simulink model "RLCbac2"  (Simulink 8.5)
settings: Solver=ode3  StartTime=0.0  StopTime=10.0  FixedStep=0.1  RelTol=1e-3
settings Model: Creator=ASUS  LastModifiedBy=ASUS
settings DataIOCC: SignalLoggingSaveFormat=Dataset
settings OptimizationCC: ExpressionDepthLimit=128
settings DebuggingCC: UnderspecifiedInitializationDetection=Simplified  MergeDetectMultiDrivingBlocksExec=error  FcnCallInpInsideContextMsg=EnableAllAsError  StateNameClashWarn=none
settings GRTTargetCC: CombineOutputUpdateFcns=on  GRTInterface=off

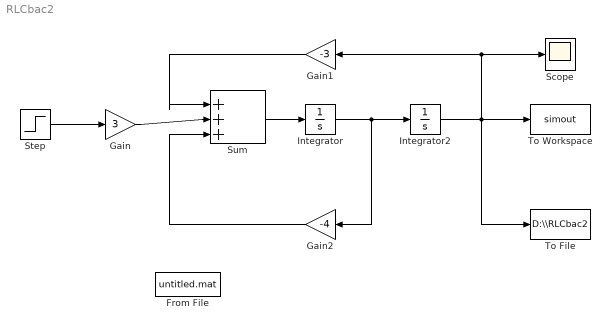
== system RLCbac2 ==
  From File : FromFile  SampleTime=0
  Gain : Gain  Gain=3
  Gain1 : Gain  Gain=-3
  Gain2 : Gain  Gain=-4
  Integrator : Integrator
  Integrator2 : Integrator
  Scope : Scope
  Step : Step  SampleTime=0
  Sum : Sum  Inputs=|+++
  To File : ToFile  Filename=D:\\RLCbac2
  To Workspace : ToWorkspace  VariableName=simout  SampleTime=-1
  wires:
  Sum/1 -> Integrator/1
  Integrator/1 -> Gain2/1, Integrator2/1
  Integrator2/1 -> To File/1, Gain1/1, Scope/1, To Workspace/1
  Gain2/1 -> Sum/3
  Step/1 -> Gain/1
  Gain/1 -> Sum/2
  Gain1/1 -> Sum/1
